simulink model "bpsk_phase"  (R2015b)
settings: Solver=VariableStepAuto  StartTime=0.0  StopTime=(12+40*7+8)*8*4-1  RelTol=1e-3
undefined symbols (not defined in the file or in its folder): jsin, K1, K2, rcosine
libraries: simulink x1
settings Model: Creator=coltmt  LastModifiedBy=coltmt

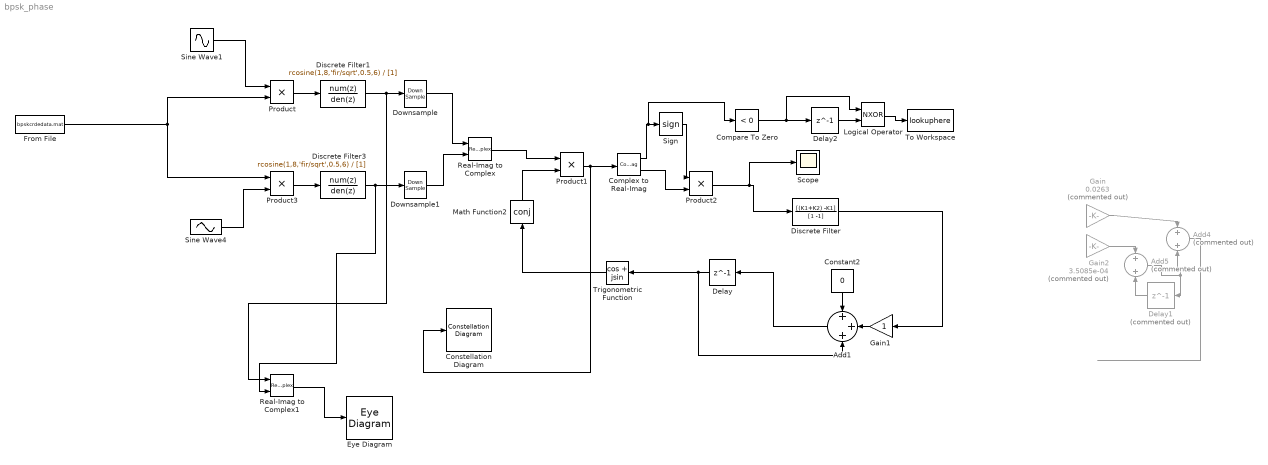
== system bpsk_phase ==
  Add1 : Sum  Inputs=+++
  Add4 : Sum  Commented=on
  Add5 : Sum  Commented=on
  Compare To Zero : simulink/Logic and Bit Operations/Compare To Zero  relop=<  OutDataTypeStr=boolean
  Complex to Real-Imag : ComplexToRealImag
  Constant2 : Constant  Value=0
  Constellation Diagram : ConstellationDiagram
  Delay : Delay  DelayLength=1
  Delay1 : Delay  Commented=on  DelayLength=1
  Delay2 : Delay  DelayLength=1  InputProcessing=Inherited
  Discrete Filter : DiscreteFilter  Numerator=[(K1+K2) -K1]  Denominator=[1 -1]
  Discrete Filter1 : DiscreteFilter  Numerator=rcosine(1,8,'fir/sqrt',0.5,6)  Denominator=[1]
  Discrete Filter3 : DiscreteFilter  Numerator=rcosine(1,8,'fir/sqrt',0.5,6)  Denominator=[1]
  Downsample : DownSample  N=8  InputProcessing=Inherited (this choice will be removed - see release notes)  RateOptions=Allow multirate processing
  Downsample1 : DownSample  N=8  InputProcessing=Inherited (this choice will be removed - see release notes)  RateOptions=Allow multirate processing
  Eye Diagram : EyeDiagram
  From File : FromFile  FileName=bpskcrdedata.mat
  Gain : Gain  Commented=on  Gain=0.0263
  Gain1 : Gain
  Gain2 : Gain  Commented=on  Gain=3.5085e-04
  Logical Operator : Logic  Operator=NXOR  AllPortsSameDT=off  OutDataTypeStr=boolean
  Math Function2 : Math  Operator=conj  SaturateOnIntegerOverflow=on
  Product{,1..3} (4 alike) : Product
  Real-Imag to Complex : RealImagToComplex
  Real-Imag to Complex1 : RealImagToComplex
  Scope : Scope
  Sign : Signum
  Sine Wave1 : Sin  Amplitude=sqrt(2)  Frequency=.2*2*pi  Phase=pi/2  SampleTime=1
  Sine Wave4 : Sin  Amplitude=-sqrt(2)  Frequency=.2*2*pi  SampleTime=1
  To Workspace : ToWorkspace  VariableName=lookuphere  SampleTime=-1
      settings: Save2DSignal=2-D array (concatenate along first dimension)
  Trigonometric Function : Trigonometry  Operator=cos + jsin
  wires:
  Constant2/1 -> Add1/1
  Add1/1 -> Delay/1
  Delay/1 -> Trigonometric Function/1, Add1/3
  Math Function2/1 -> Product1/2
  Gain1/1 -> Add1/2
  Trigonometric Function/1 -> Math Function2/1
  Sine Wave1/1 -> Product/1
  Sine Wave4/1 -> Product3/2
  Product/1 -> Discrete Filter1/1
  Product3/1 -> Discrete Filter3/1
  Discrete Filter1/1 -> Real-Imag to Complex1/1, Downsample/1
  From File/1 -> Product/2, Product3/1
  Real-Imag to Complex/1 -> Product1/1
  Downsample1/1 -> Real-Imag to Complex/2
  Downsample/1 -> Real-Imag to Complex/1
  Product1/1 -> Constellation Diagram/1, Complex to Real-Imag/1
  Complex to Real-Imag/1 -> Compare To Zero/1, Sign/1
  Sign/1 -> Product2/1
  Complex to Real-Imag/2 -> Product2/2
  Discrete Filter3/1 -> Real-Imag to Complex1/2, Downsample1/1
  Real-Imag to Complex1/1 -> Eye Diagram/1
  Gain/1 -> Add4/1
  Delay1/1 -> Add5/2
  Add5/1 -> Delay1/1, Add4/2
  Gain2/1 -> Add5/1
  Add4/1 -> ?
  Discrete Filter/1 -> Gain1/1
  Product2/1 -> Scope/1, Discrete Filter/1
  Logical Operator/1 -> To Workspace/1
  Delay2/1 -> Logical Operator/2
  Compare To Zero/1 -> Logical Operator/1, Delay2/1
